simulink model "Experiment_2_cs"  (Simulink 8.4)
settings: Solver=ode5  SolverMode=SingleTasking  StartTime=0.0  StopTime=inf  FixedStep=1/100  RelTol=1e-3
model workspace (MAT data in the model file):
  mbox_table : struct (value not decoded)
  model_closed = 0
  sim_status : num (value not decoded)
PreLoadFcn:
  | mbxruntime.callbacks.PreLoadFcn(bdroot);
PostLoadFcn:
  | mbxruntime.callbacks.PostLoadFcn(bdroot);
InitFcn:
  | mbxruntime.callbacks.InitFcn(bdroot);
StartFcn:
  | mbxruntime.callbacks.StartFcn(bdroot);
StopFcn:
  | mbxruntime.callbacks.StopFcn(bdroot);
undefined symbols (not defined in the file or in its folder): dfreq, gray, InitImageOutputDir, Rec, SDTV, strel, warningInitialVelocity, x0
libraries: simulink x43, PreScanSimulinkLibrary x19, visiontextngfix x15, simulink_extras x11, visionconversions x3, PreScanUsefulBlocks x3, visionsinks x2, visionstatistics x1, visionmorphops x1, visionanalysis x1
(part 1 of 8)
CloseFcn:
  | mbxruntime.callbacks.CloseFcn(bdroot);
settings Model: Creator=PRESCAN  LastModifiedBy=vj-admin
settings OptimizationCC: InitFltsAndDblsToZero=on
settings DebuggingCC: SaveWithParameterizedLinksMsg=none  SignalResolutionControl=TryResolveAllWithWarning  SolverPrmCheckMsg=none  MultiTaskDSMMsg=warning  MultiTaskCondExecSysMsg=none
settings ModelReferenceCC: UpdateModelReferenceTargets=IfOutOfDate
settings SFSimCC: SimParseCustomCode=off
settings SFSimCC: SimCustomHeaderCode=|
  | #include "prescan_collisiondetection_data.h"
  | #include "prescan.h"
  | #include "prescan_platform.h"
  | #include "prescan_v2x_data.h"
settings RTWCC: IncludeERTFirstTime=on
settings GRTTargetCC: TargetFcnLib=ansi_tfl_tmw.mat

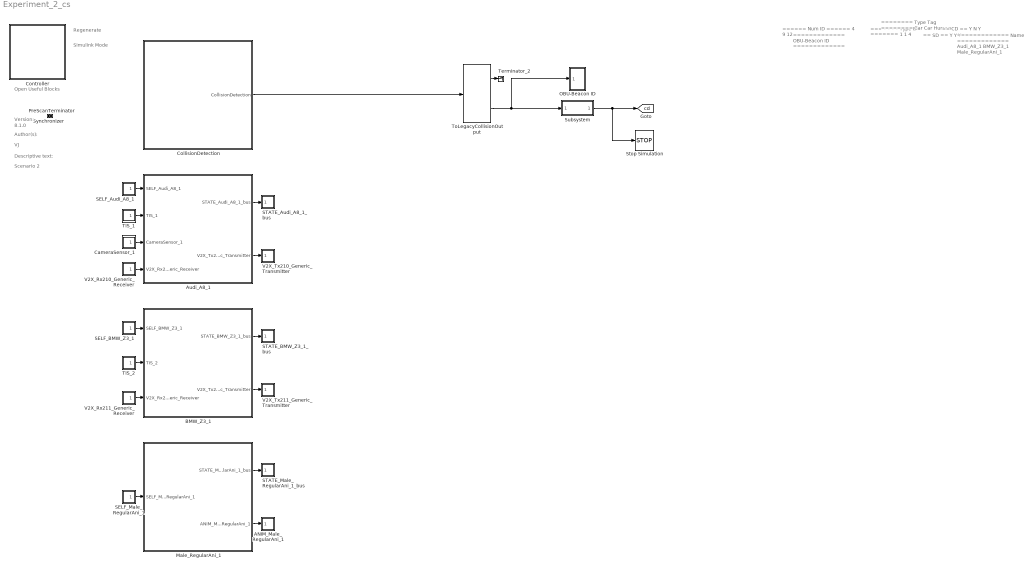
== system Experiment_2_cs ==
  note: Regenerate
  note: Simulink Mode
  note: Open Useful Blocks
  note: 8.1.0
  note: Version:
  note: Author(s):
  note: VJ
  note: Descriptive text:
  note: Scenario 2
  note: ======
      | Num ID
      | ======
      | 4
      | 9
      | 12
  note: =============
      | OBU-Beacon ID
      | =============
  note: =======
      | Type ID
      | =======
      | 1
      | 1
      | 4
  note: ========
      | Type Tag
      | ========
      | Car
      | Car
      | Human
  note: ==
      | SD
      | ==
      | Y
      | Y
      | Y
  note: ==
      | CD
      | ==
      | Y
      | N
      | Y
  note: =============
      | Name
      | =============
      | Audi_A8_1
      | BMW_Z3_1
      | Male_RegularAni_1
  ANIM_Male_RegularAni_1 : Subsystem  Tag=actuator/AnimationOutport  Priority=0  LoadFcn=load('PreScanAnimActuatorData.mat')  Variant=on  OverrideUsingVariant=on  mask(PreScan Sink Block: State Animation){}
      mask help: The Human Animation port allows the human to walk, run or bend
      settings: OpenFcn=open_system([gcb '/ENABLED/Actuator'],'mask')
      mask Help: eval('openHelp(239)')
      mask Display: image(imread('HumanAnimated.jpg'))
  Audi_A8_1 : Subsystem  Tag=WorldObjectSubSystem  InitFcn=UniqueId = '109';  Variant=on  OverrideUsingVariant=on
      mask init:
      | imagePath=which('Audi_A8.jpg');
      settings: OpenFcn=open_system([gcb '/ENABLED'])
      mask Display: image(imread(imagePath));color('white');text(0,0,' ID=4\n')
  BMW_Z3_1 : Subsystem  Tag=WorldObjectSubSystem  InitFcn=UniqueId = '112';  Variant=on  OverrideUsingVariant=on
      mask init:
      | imagePath=which('BMW_Z3.jpg');
      settings: OpenFcn=open_system([gcb '/ENABLED'])
      mask Display: image(imread(imagePath));color('white');text(0,0,' ID=9\n')
  CameraSensor_1 : Subsystem  Tag=sensor/Camera/CameraSensor  Priority=3  Variant=on  OverrideUsingVariant=on  mask(PreScan Source Block: Camera Sensor){}
      mask help: The Camera Sensor provides a color or monochrome image.
      settings: OpenFcn=open_system([gcb '/ENABLED/Sensor'],'mask')
      mask Help: eval('openHelp(457)')
      mask Display: image(imread('CameraSensor.png'))
  CollisionDetection : Subsystem  Tag=sensor/CollisionDetection  Priority=3  LoadFcn=load('PrescanCollisionDetectionData.mat');load('PrescanCollisionDetectionMessage.mat')  Variant=on  OverrideUsingVariant=on  mask(PreScan Source Block: CollisionDetection){}
      mask help: Collision Detection can be used to detect collisions between PreScan components. For Collision Detection the actual component shape is taken into account, so it is not a bounding box approach.
      settings: OpenFcn=open_system([gcb '/ENABLED/Sensor'],'mask')
      mask Help: eval('openHelp(811)')
      mask Display: image(imread('crash.jpg'))
  Controller : Subsystem  Description=FA0A96F99A880E53F0BFF9FE52303144F19899D73F656CE8BF47A1C0F136E2DD  Priority=-1  LoadFcn=load PreScanControllerData  mask(PreScan Simulation Controller){prescanversion='8.1.0', ModelReferencing=off, TimeStep=1/100, ControlMode=0, PreScanExecutionMode=on, ControllerCount=0, ControllerIndex=0, ControllerOptions=''}
      mask prompts: prescanversion "PreScan Version"; ModelReferencing "Use Model Referencing"; TimeStep "Upload Period [s]"; ControlMode "Control Mode"; PreScanExecutionMode "Execution Mode"; ControllerCount "Controller Count"; ControllerIndex "Controller Index"; ControllerOptions "Controller Options"
      mask help:
      | Please do not remove this block from the compilation sheet,
      | as it connects the model to the PreScan environment.
      mask init:
      | model = bdroot(gcb);
      | ExperimentFile = mbxruntime.findExperimentFile(model);
      | 
      | [d1, d2, d3, prescandata] = prescan_Settings();
      | ModelDepo = fullfile(prescandata,'ModelDepo'); 
      | 
      | RTmode = 0;
      | actors = find_system(model,'SearchDepth', 1,'LookUnderMasks', 'all','Tag','WorldObjectSubSystem');
      | for ii=1:length(actors)
      |     actormode = get_param(actors{ii},'OverrideUsingVariant');
      |     if strcmpi(actormode,'off')
      |         RTmode = 1;
      |     end
      | end
      | 
      | SimulationMode = get_param(bdroot,'SimulationMode');
      | if strcmp(SimulationMode, 'rapid-accelerator')
      |     SimulationMode = 'external';
      | end
      | TargetName = get_param(bdroot,'SystemTargetFile');
      settings: ModelCloseFcn=assignin('base',['model_closed_' bdroot],true);
      mask Help: eval('openHelp(812)')
      mask Display: image(imread('prescanlogo.ico'))
  Male_RegularAni_1 : Subsystem  Tag=WorldObjectSubSystem  InitFcn=UniqueId = '116';  Variant=on  OverrideUsingVariant=on
      mask init:
      | imagePath=which('Male_RegularAni.jpg');
      settings: OpenFcn=open_system([gcb '/ENABLED'])
      mask Display: image(imread(imagePath));color('white');text(0,0,' ID=12\n')
  OBU-Beacon ID : Subsystem  Tag=Scope Collision Detections
      settings: DeleteFcn=PreScanBlockDeleteFcn;
      settings: OpenFcn=|
      | blockname=[get_param(gcb,'Parent'),'/',get_param(gcb,'Name')];
      | subblockname=[blockname,'/Collision Detections'];
      | open_system(subblockname);
      | close_system(blockname);
      mask Display:
      | plot([0.5 9.5 9.5 0.5 0.5],[5 5 9 9 5])
      | plot(0,0)
      | plot(10,10)
      | text(0,1,'P+')
  PreScanTerminator : Subsystem  Tag=PreScanTerminator  Priority=999  LoadFcn=load PrescanTerminatorData  mask(PreScan Simulation Terminator){TimeStep=1/100}
      mask prompts: TimeStep "Upload Period [s]"
      mask help:
      | Please do not remove this block from the compilation sheet as it
      | connects the model to the PreScan environment.
      mask Help: eval('openHelp(812)')
      mask Display: image(imread('prescanlogo.ico'))
  SELF_Audi_A8_1 : Subsystem  Tag=sensor/SelfPort  Priority=3  LoadFcn=load('PreScanSelfSensorData.mat')  Variant=on  OverrideUsingVariant=on  mask(PreScan Source Block: SELF){}
      mask help:
      | The SELF port shows (state) information of the actor itself. The outputs are position in the experiment's axis system and the GPS coordinates, and the object's absolute velocity and compass heading.
      |
      | For more information, please click Help.
      settings: OpenFcn=open_system([gcb '/ENABLED/Sensor'],'mask')
      mask Help: eval('openHelp(462)')
      mask Display: image(imread('GPS.png'))
  SELF_BMW_Z3_1 : Subsystem  Tag=sensor/SelfPort  Priority=3  LoadFcn=load('PreScanSelfSensorData.mat')  Variant=on  OverrideUsingVariant=on  mask(PreScan Source Block: SELF){}
      mask help:
      | The SELF port shows (state) information of the actor itself. The outputs are position in the experiment's axis system and the GPS coordinates, and the object's absolute velocity and compass heading.
      |
      | For more information, please click Help.
      settings: OpenFcn=open_system([gcb '/ENABLED/Sensor'],'mask')
      mask Help: eval('openHelp(462)')
      mask Display: image(imread('GPS.png'))
  SELF_Male_RegularAni_1 : Subsystem  Tag=sensor/SelfPort  Priority=3  LoadFcn=load('PreScanSelfSensorData.mat')  Variant=on  OverrideUsingVariant=on  mask(PreScan Source Block: SELF){}
      mask help:
      | The SELF port shows (state) information of the actor itself. The outputs are position in the experiment's axis system and the GPS coordinates, and the object's absolute velocity and compass heading.
      |
      | For more information, please click Help.
      settings: OpenFcn=open_system([gcb '/ENABLED/Sensor'],'mask')
      mask Help: eval('openHelp(462)')
      mask Display: image(imread('GPS.png'))
  STATE_Audi_A8_1_bus : Subsystem  Tag=actuator/StatePort  Priority=0  LoadFcn=load('PreScanStateActuatorData.mat')  Variant=on  OverrideUsingVariant=on  mask(PreScan Sink Block: State){}
      mask help:
      | The Actor State contains a vector signal of size (9x1), containing the following signals:
      |
      | -  Position    	(x,y,z)             	[m]
      | -  Velocity    	(vx,vy,vz)         	[m/s]
      | -  Angles       	(Roll, Pitch, Yaw)	[rad]
      |
      | The Actor state is defined in the global axis system.
      | The state is superponed on the Initial position defined in the GUI.
      |
      | For more information, please click Help.
      settings: OpenFcn=open_system([gcb '/ENABLED/Actuator'],'mask')
      mask Help: eval('openHelp(222)')
      mask Display: image(imread('State.png'))
  STATE_BMW_Z3_1_bus : Subsystem  Tag=actuator/StatePort  Priority=0  LoadFcn=load('PreScanStateActuatorData.mat')  Variant=on  OverrideUsingVariant=on  mask(PreScan Sink Block: State){}
      mask help:
      | The Actor State contains a vector signal of size (9x1), containing the following signals:
      |
      | -  Position    	(x,y,z)             	[m]
      | -  Velocity    	(vx,vy,vz)         	[m/s]
      | -  Angles       	(Roll, Pitch, Yaw)	[rad]
      |
      | The Actor state is defined in the global axis system.
      | The state is superponed on the Initial position defined in the GUI.
      |
      | For more information, please click Help.
      settings: OpenFcn=open_system([gcb '/ENABLED/Actuator'],'mask')
      mask Help: eval('openHelp(222)')
      mask Display: image(imread('State.png'))
  STATE_Male_RegularAni_1_bus : Subsystem  Tag=actuator/StatePort  Priority=0  LoadFcn=load('PreScanStateActuatorData.mat')  Variant=on  OverrideUsingVariant=on  mask(PreScan Sink Block: State){}
      mask help:
      | The Actor State contains a vector signal of size (9x1), containing the following signals:
      |
      | -  Position    	(x,y,z)             	[m]
      | -  Velocity    	(vx,vy,vz)         	[m/s]
      | -  Angles       	(Roll, Pitch, Yaw)	[rad]
      |
      | The Actor state is defined in the global axis system.
      | The state is superponed on the Initial position defined in the GUI.
      |
      | For more information, please click Help.
      settings: OpenFcn=open_system([gcb '/ENABLED/Actuator'],'mask')
      mask Help: eval('openHelp(222)')
      mask Display: image(imread('State.png'))
  Stop Simulation : Stop
  Subsystem : Subsystem
      mask Display: fprintf('CD');
  Synchronizer : Subsystem  Tag=PreScanSynchronizer  Priority=1  LoadFcn=load PrescanSynchronizeData  mask(PreScan Simulation Core Block){TimeStep=1/100}
      mask prompts: TimeStep "Timestep [s]"
      mask help:
      | Please do not remove this block from the PreScan compilation sheet,
      | as it contains essential configuration parameters for a PreScan simulation.
      settings: DeleteFcn=PreScanBlockDeleteFcn;
      mask Display: image(imread('prescanlogo.ico'))
  TIS_1 : Subsystem  Tag=sensor/TIS  Priority=3  LoadFcn=load('PrescanScannerSensorData.mat');load('PrescanScannerSensorMessage.mat')  Variant=on  OverrideUsingVariant=on  mask(PreScan Source Block: Technology Independent Sensor (TIS)){}
      mask help:
      | The Technology Independent Sensor (TIS) provides a sensor with all sensor-related influence factors (like noise, drift and accuracy) without being technology specific (like radar and lidar). The TIS detects the closest point on the geometry of an object.
      |
      | For more information, please click Help.
      settings: OpenFcn=open_system([gcb '/ENABLED/Sensor'],'mask')
      mask Help: eval('openHelp(449)')
      mask Display: image(imread('TIS.png'))
  TIS_2 : Subsystem  Tag=sensor/TIS  Priority=3  LoadFcn=load('PrescanScannerSensorData.mat');load('PrescanScannerSensorMessage.mat')  Variant=on  OverrideUsingVariant=on  mask(PreScan Source Block: Technology Independent Sensor (TIS)){}
      mask help:
      | The Technology Independent Sensor (TIS) provides a sensor with all sensor-related influence factors (like noise, drift and accuracy) without being technology specific (like radar and lidar). The TIS detects the closest point on the geometry of an object.
      |
      | For more information, please click Help.
      settings: OpenFcn=open_system([gcb '/ENABLED/Sensor'],'mask')
      mask Help: eval('openHelp(449)')
      mask Display: image(imread('TIS.png'))
  Terminator_2 : Terminator
  ToLegacyCollisionOutput : PreScanUsefulBlocks/ToLegacyCollisionOutput
  V2X_Rx210_Generic_Receiver : Subsystem  Tag=sensor/plugin/sfun_V2X_Generic_Receiver  Priority=3  Variant=on  OverrideUsingVariant=on  mask(V2X Generic Receiver Block){}
      mask help: V2X Block receiving a Generic message
      settings: OpenFcn=open_system([gcb '/ENABLED/Sensor'],'mask')
      mask Help: eval('openHelp()')
      mask Display: image(imread('V2XR_grayscale.png'))
  V2X_Rx211_Generic_Receiver : Subsystem  Tag=sensor/plugin/sfun_V2X_Generic_Receiver  Priority=3  Variant=on  OverrideUsingVariant=on  mask(V2X Generic Receiver Block){}
      mask help: V2X Block receiving a Generic message
      settings: OpenFcn=open_system([gcb '/ENABLED/Sensor'],'mask')
      mask Help: eval('openHelp()')
      mask Display: image(imread('V2XR_grayscale.png'))
  V2X_Tx210_Generic_Transmitter : Subsystem  Tag=actuator/plugin/sfun_V2X_Generic_Transmitter  Priority=0  Variant=on  OverrideUsingVariant=on  mask(V2X Generic Transmitter Block){}
      mask help: V2X Block transmitting a Generic message
      settings: OpenFcn=open_system([gcb '/ENABLED/Actuator'],'mask')
      mask Help: eval('openHelp()')
      mask Display: image(imread('V2XT_grayscale.png'))
  V2X_Tx211_Generic_Transmitter : Subsystem  Tag=actuator/plugin/sfun_V2X_Generic_Transmitter  Priority=0  Variant=on  OverrideUsingVariant=on  mask(V2X Generic Transmitter Block){}
      mask help: V2X Block transmitting a Generic message
      settings: OpenFcn=open_system([gcb '/ENABLED/Actuator'],'mask')
      mask Help: eval('openHelp()')
      mask Display: image(imread('V2XT_grayscale.png'))
  tag scope: cd=global
  wires:
  CollisionDetection/1(CollisionDetection) -> ToLegacyCollisionOutput/1
  Subsystem/1(cd_out) -> Stop Simulation/1, [cd]
  ToLegacyCollisionOutput/2 -> Subsystem/1(cd_in), OBU-Beacon ID/1(In1)
  ToLegacyCollisionOutput/1 -> Terminator_2/1
  Audi_A8_1/1(STATE_Audi_A8_1_bus) -> STATE_Audi_A8_1_bus/1(STATE_Audi_A8_1_bus)
  SELF_Audi_A8_1/1(SELF_Audi_A8_1) -> Audi_A8_1/1(SELF_Audi_A8_1)
  TIS_1/1(TIS_1) -> Audi_A8_1/2(TIS_1)
  CameraSensor_1/1(CameraSensor_1) -> Audi_A8_1/3(CameraSensor_1)
  Audi_A8_1/2(V2X_Tx210_Generic_Transmitter) -> V2X_Tx210_Generic_Transmitter/1(V2X_Tx210_Generic_Transmitter)
  V2X_Rx210_Generic_Receiver/1(V2X_Rx210_Generic_Receiver) -> Audi_A8_1/4(V2X_Rx210_Generic_Receiver)
  BMW_Z3_1/1(STATE_BMW_Z3_1_bus) -> STATE_BMW_Z3_1_bus/1(STATE_BMW_Z3_1_bus)
  SELF_BMW_Z3_1/1(SELF_BMW_Z3_1) -> BMW_Z3_1/1(SELF_BMW_Z3_1)
  TIS_2/1(TIS_2) -> BMW_Z3_1/2(TIS_2)
  BMW_Z3_1/2(V2X_Tx211_Generic_Transmitter) -> V2X_Tx211_Generic_Transmitter/1(V2X_Tx211_Generic_Transmitter)
  V2X_Rx211_Generic_Receiver/1(V2X_Rx211_Generic_Receiver) -> BMW_Z3_1/3(V2X_Rx211_Generic_Receiver)
  Male_RegularAni_1/1(STATE_Male_RegularAni_1_bus) -> STATE_Male_RegularAni_1_bus/1(STATE_Male_RegularAni_1_bus)
  Male_RegularAni_1/2(ANIM_Male_RegularAni_1) -> ANIM_Male_RegularAni_1/1(ANIM_Male_RegularAni_1)
  SELF_Male_RegularAni_1/1(SELF_Male_RegularAni_1) -> Male_RegularAni_1/1(SELF_Male_RegularAni_1)

== system Experiment_2_cs/ANIM_Male_RegularAni_1 ==
  ANIM_Male_RegularAni_1 : Inport  Tag=inport/AnimationOutport  OutDataTypeStr=Bus: PRESCAN_ANIMACTUATORDATA  PortDimensions=1  SampleTime=1/100  BusOutputAsStruct=on
  DISABLED : Subsystem  VariantControl=off
  ENABLED : Subsystem  VariantControl=on

== system Experiment_2_cs/Audi_A8_1 ==
  SELF_Audi_A8_1 : Inport  Tag=inport/SelfPort  OutDataTypeStr=Bus: PRESCAN_SELFSENSORDATA  PortDimensions=1  SampleTime=1/100  BusOutputAsStruct=on
  TIS_1 : Inport  Tag=inport/TIS  Port=2  OutDataTypeStr=Bus: PRESCAN_SCANNERSENSOR_MESSAGE  PortDimensions=3  SampleTime=1/50  BusOutputAsStruct=on
  CameraSensor_1 : Inport  Tag=inport/Camera/CameraSensor  Port=3  OutDataTypeStr=uint8  SampleTime=1/50  BusOutputAsStruct=on
  V2X_Rx210_Generic_Receiver : Inport  Tag=inport/plugin/sfun_V2X_Generic_Receiver  Port=4  BusOutputAsStruct=on
  DISABLED : Subsystem  VariantControl=off
  ENABLED : Subsystem  VariantControl=on
  STATE_Audi_A8_1_bus : Outport  Tag=outport/StatePort  OutDataTypeStr=Bus: PRESCAN_STATEACTUATORDATA  PortDimensions=1  SampleTime=1/100
  V2X_Tx210_Generic_Transmitter : Outport  Tag=outport/plugin/sfun_V2X_Generic_Transmitter  Port=2

== system Experiment_2_cs/BMW_Z3_1 ==
  SELF_BMW_Z3_1 : Inport  Tag=inport/SelfPort  OutDataTypeStr=Bus: PRESCAN_SELFSENSORDATA  PortDimensions=1  SampleTime=1/100  BusOutputAsStruct=on
  TIS_2 : Inport  Tag=inport/TIS  Port=2  OutDataTypeStr=Bus: PRESCAN_SCANNERSENSOR_MESSAGE  PortDimensions=3  SampleTime=1/50  BusOutputAsStruct=on
  V2X_Rx211_Generic_Receiver : Inport  Tag=inport/plugin/sfun_V2X_Generic_Receiver  Port=3  BusOutputAsStruct=on
  DISABLED : Subsystem  VariantControl=off
  ENABLED : Subsystem  VariantControl=on
  STATE_BMW_Z3_1_bus : Outport  Tag=outport/StatePort  OutDataTypeStr=Bus: PRESCAN_STATEACTUATORDATA  PortDimensions=1  SampleTime=1/100
  V2X_Tx211_Generic_Transmitter : Outport  Tag=outport/plugin/sfun_V2X_Generic_Transmitter  Port=2

== system Experiment_2_cs/CameraSensor_1 ==
  DISABLED : Subsystem  VariantControl=off
  ENABLED : Subsystem  VariantControl=on
  CameraSensor_1 : Outport  Tag=outport/Camera/CameraSensor  OutDataTypeStr=uint8  SampleTime=1/50

== system Experiment_2_cs/CollisionDetection ==
  DISABLED : Subsystem  VariantControl=off
  ENABLED : Subsystem  VariantControl=on
  CollisionDetection : Outport  Tag=outport/CollisionDetection  OutDataTypeStr=Bus: PRESCAN_COLLISIONDETECTION_MESSAGE  PortDimensions=5  SampleTime=1/100

== system Experiment_2_cs/Controller ==
  Terminator : Terminator
  sfun_Controller : S-Function  FunctionName=sfun_Controller  Parameters=SParameter1, SParameter2, SParameter3, SParameter4, SParameter5, SParameter6, SParameter7, SParameter8, SParameter9, SParameter10, SampleTime  EnableBusSupport=off  mask(Legacy Function){SFunctionSpec=void prescan_outputFcn(void** work1, PRESCAN_CONTROLLERDATA y1[1]), SParameter1=uint8([ExperimentFile 0]), SParameter2=uint8([ModelDepo 0]), SParameter3=uint8([ControllerOptions 0]), SParameter4=RTmode, SParameter5=PreScanExecutionMode, SParameter6=ControlMode, SParameter7=ControllerCount, SParameter8=ControllerIndex, SParameter9=uint8([SimulationMode 0]), SParameter10=uint8([TargetName 0]), SampleTime=TimeStep, ShowSpec=on}
      mask prompts: SParameter1 "P1:"; SParameter2 "P2:"; SParameter3 "P3:"; SParameter4 "P4:"; SParameter5 "P5:"; SParameter6 "P6:"; SParameter7 "P7:"; SParameter8 "P8:"; SParameter9 "P9:"; SParameter10 "P10:"; SampleTime "Sample time (-1 for inherited):"; ShowSpec "Display function specification"
      mask help:
      | This block allows you to call the legacy functions specified by the following Legacy Code Tool definition:
      | def.SFunctionName = 'sfun_Controller';
      | def.OutputFcnSpec = 'void prescan_outputFcn(void** work1, PRESCAN_CONTROLLERDATA y1[1])';
      | def.StartFcnSpec = 'void prescan_startFcn(void ** work1, uint8 p1[], uint8 p2[], uint8 p3[], double p4, double p5, double p6, double p7, double p8, uint8 p9[], uint8 p10[])';
      | def.TerminateFcnSpec = 'void prescan_terminateFcn(void** work1)';
      | def.HeaderFiles = {'prescan_controller_data.h', 'prescan_SFunLibrary.h', 'prescan_LogHandler.h', 'prescan_CreateLogHandler.h', 'prescan_ErrorHandler.h', 'prescan_CreateErrorHandler.h', 'prescan_modify.h', 'ModuleDLL.h'};
      | def.SourceFiles = {'prescan_MexLogHandler.cpp', 'prescan_SimStructErrorHandler.cpp', 'prescan_LogHandler.cpp', 'prescan_ErrorHandler.cpp', 'prescan_Modify.cpp'};
      | def.HostLibFiles = {'sensorinterfaced.lib'};
      | def.TargetLibFiles = {'sensorinterfaced.so'};
      | def.IncPaths = {'.', 'C:\projects\prescan\rt_vislibrary\vis\..\pimp\include\sensors\InterfaceRTW'};
      | def.SrcPaths = {'C:\projects\prescan\rt_vislibrary\vis\..\pimp\include\sensors\InterfaceRTW', 'C:\projects\prescan\rt_vislibrary\vis\..\pimp\include\sensors\InterfaceRTW\ccurrt'};
      | def.LibPaths = {'C:\\projects\\prescan\\vislibrary_build\lib'};
      | def.SampleTime = 'parameterized';
      mask Help: <p>This block was generated automatically by the Legacy Code Tool. For detailed help on this tool, call<a href="matlab:legacy_code('help')"> legacy_code('help')</a>.</p>
      mask Callback ShowSpec:
      | if strcmp(get_param(gcbh, 'ShowSpec'), 'on')
      |   set_param(gcbh, 'MaskDisplay', sprintf('fprintf(''%s'');', get_param(gcbh, 'SFunctionSpec')));
      | else
      |   set_param(gcbh, 'MaskDisplay', sprintf('fprintf(''%s'');', get_param(gcbh, 'FunctionName')));
      | end
      mask Display: fprintf('void prescan_outputFcn(void** work1, PRESCAN_CONTROLLERDATA y1[1])');
  wires:
  sfun_Controller/1 -> Terminator/1

== system Experiment_2_cs/Male_RegularAni_1 ==
  SELF_Male_RegularAni_1 : Inport  Tag=inport/SelfPort  OutDataTypeStr=Bus: PRESCAN_SELFSENSORDATA  PortDimensions=1  SampleTime=1/100  BusOutputAsStruct=on
  DISABLED : Subsystem  VariantControl=off
  ENABLED : Subsystem  VariantControl=on
  STATE_Male_RegularAni_1_bus : Outport  Tag=outport/StatePort  OutDataTypeStr=Bus: PRESCAN_STATEACTUATORDATA  PortDimensions=1  SampleTime=1/100
  ANIM_Male_RegularAni_1 : Outport  Tag=outport/AnimationOutport  Port=2  OutDataTypeStr=Bus: PRESCAN_ANIMACTUATORDATA  PortDimensions=1  SampleTime=1/100

== system Experiment_2_cs/OBU-Beacon ID ==
  In1 : Inport
  Collision Detections : Scope  NumInputPorts=5
      settings: YMin=0~0~0~0~0  YMax=10~10~10~10~10  SaveName=ScopeData2
  Demux2 : Demux  Outputs=5
  wires:
  In1/1 -> Demux2/1
  Demux2/5 -> Collision Detections/5
  Demux2/4 -> Collision Detections/4
  Demux2/3 -> Collision Detections/3
  Demux2/2 -> Collision Detections/2
  Demux2/1 -> Collision Detections/1

== system Experiment_2_cs/PreScanTerminator ==
  Terminator : Terminator
  sfun_Terminator : S-Function  FunctionName=sfun_Terminator  Parameters=SampleTime  EnableBusSupport=off  mask(Legacy Function){SFunctionSpec=void prescan_terminator_outputFcn(void ** work1, PRESCAN_TERMINATORDATA y1[1]), SampleTime=TimeStep, ShowSpec=on}
      mask prompts: SampleTime "Sample time (-1 for inherited):"; ShowSpec "Display function specification"
      mask help:
      | This block allows you to call the legacy functions specified by the following Legacy Code Tool definition:
      | def.SFunctionName = 'sfun_Terminator';
      | def.OutputFcnSpec = 'void prescan_terminator_outputFcn(void ** work1, PRESCAN_TERMINATORDATA y1[1])';
      | def.StartFcnSpec = 'void prescan_terminator_startFcn(void ** work1)';
      | def.TerminateFcnSpec = 'void prescan_terminator_terminateFcn(void ** work1)';
      | def.HeaderFiles = {'prescan_terminator_data.h'};
      | def.HostLibFiles = {'sensorinterfaced.lib'};
      | def.IncPaths = {'src', 'C:\prescandev\vislibrary\vis\..\pimp\include\sensors\InterfaceRTW'};
      | def.SrcPaths = {'src'};
      | def.LibPaths = {'C:\\prescandev\\vislibrary_build\lib'};
      | def.SampleTime = 'parameterized';
      | def.Options.language = 'C++';
      mask Help: <p>This block was generated automatically by the Legacy Code Tool. For detailed help on this tool, call<a href="matlab:legacy_code('help')"> legacy_code('help')</a>.</p>
      mask Callback ShowSpec:
      | if strcmp(get_param(gcbh, 'ShowSpec'), 'on')
      |   set_param(gcbh, 'MaskDisplay', sprintf('fprintf(''%s'');', get_param(gcbh, 'SFunctionSpec')));
      | else
      |   set_param(gcbh, 'MaskDisplay', sprintf('fprintf(''%s'');', get_param(gcbh, 'FunctionName')));
      | end
      mask Display: fprintf('void prescan_terminator_outputFcn(void ** work1, PRESCAN_TERMINATORDATA y1[1])');
  wires:
  sfun_Terminator/1 -> Terminator/1

== system Experiment_2_cs/SELF_Audi_A8_1 ==
  DISABLED : Subsystem  VariantControl=off
  ENABLED : Subsystem  VariantControl=on
  SELF_Audi_A8_1 : Outport  Tag=outport/SelfPort  OutDataTypeStr=Bus: PRESCAN_SELFSENSORDATA  PortDimensions=1  SampleTime=1/100

== system Experiment_2_cs/SELF_BMW_Z3_1 ==
  DISABLED : Subsystem  VariantControl=off
  ENABLED : Subsystem  VariantControl=on
  SELF_BMW_Z3_1 : Outport  Tag=outport/SelfPort  OutDataTypeStr=Bus: PRESCAN_SELFSENSORDATA  PortDimensions=1  SampleTime=1/100

== system Experiment_2_cs/SELF_Male_RegularAni_1 ==
  DISABLED : Subsystem  VariantControl=off
  ENABLED : Subsystem  VariantControl=on
  SELF_Male_RegularAni_1 : Outport  Tag=outport/SelfPort  OutDataTypeStr=Bus: PRESCAN_SELFSENSORDATA  PortDimensions=1  SampleTime=1/100

== system Experiment_2_cs/STATE_Audi_A8_1_bus ==
  STATE_Audi_A8_1_bus : Inport  Tag=inport/StatePort  OutDataTypeStr=Bus: PRESCAN_STATEACTUATORDATA  PortDimensions=1  SampleTime=1/100  BusOutputAsStruct=on
  DISABLED : Subsystem  VariantControl=off
  ENABLED : Subsystem  VariantControl=on

== system Experiment_2_cs/STATE_BMW_Z3_1_bus ==
  STATE_BMW_Z3_1_bus : Inport  Tag=inport/StatePort  OutDataTypeStr=Bus: PRESCAN_STATEACTUATORDATA  PortDimensions=1  SampleTime=1/100  BusOutputAsStruct=on
  DISABLED : Subsystem  VariantControl=off
  ENABLED : Subsystem  VariantControl=on

== system Experiment_2_cs/STATE_Male_RegularAni_1_bus ==
  STATE_Male_RegularAni_1_bus : Inport  Tag=inport/StatePort  OutDataTypeStr=Bus: PRESCAN_STATEACTUATORDATA  PortDimensions=1  SampleTime=1/100  BusOutputAsStruct=on
  DISABLED : Subsystem  VariantControl=off
  ENABLED : Subsystem  VariantControl=on

== system Experiment_2_cs/Subsystem ==
  cd_in : Inport
  Integer Delay : Delay  DelayLength=1  InputProcessing=Inherited
  Logical Operator : Logic  AllPortsSameDT=off  OutDataTypeStr=boolean
  cd_out : Outport
  wires:
  cd_in/1 -> Integer Delay/1, Logical Operator/1
  Logical Operator/1 -> cd_out/1
  Integer Delay/1 -> Logical Operator/2

== system Experiment_2_cs/Synchronizer ==
  Bus Selector1 : BusSelector  OutputSignals=FederateStopped
  Stop Simulation : Stop
  sfun_Synchronizer : S-Function  FunctionName=sfun_Synchronizer  Parameters=SampleTime  EnableBusSupport=off  mask(Legacy Function){SFunctionSpec=void prescan_synchronizer_outputFcn(void ** work1, PRESCAN_SYNCHRONIZEDATA y1[1]), SampleTime=TimeStep, ShowSpec=on}
      mask prompts: SampleTime "Sample time (-1 for inherited):"; ShowSpec "Display function specification"
      mask help:
      | This block allows you to call the legacy functions specified by the following Legacy Code Tool definition:
      | def.SFunctionName = 'sfun_Synchronizer';
      | def.OutputFcnSpec = 'void prescan_synchronizer_outputFcn(void ** work1, PRESCAN_SYNCHRONIZEDATA y1[1])';
      | def.StartFcnSpec = 'void prescan_synchronizer_startFcn(void ** work1)';
      | def.TerminateFcnSpec = 'void prescan_synchronizer_terminateFcn(void ** work1)';
      | def.HeaderFiles = {'prescan_synchronizer_data.h'};
      | def.HostLibFiles = {'sensorinterfaced.lib'};
      | def.IncPaths = {'src', 'C:\prescandev\vislibrary\vis\..\pimp\include\sensors\InterfaceRTW'};
      | def.SrcPaths = {'src'};
      | def.LibPaths = {'C:\\prescandev\\vislibrary_build\lib'};
      | def.SampleTime = 'parameterized';
      | def.Options.language = 'C++';
      mask Help: <p>This block was generated automatically by the Legacy Code Tool. For detailed help on this tool, call<a href="matlab:legacy_code('help')"> legacy_code('help')</a>.</p>
      mask Callback ShowSpec:
      | if strcmp(get_param(gcbh, 'ShowSpec'), 'on')
      |   set_param(gcbh, 'MaskDisplay', sprintf('fprintf(''%s'');', get_param(gcbh, 'SFunctionSpec')));
      | else
      |   set_param(gcbh, 'MaskDisplay', sprintf('fprintf(''%s'');', get_param(gcbh, 'FunctionName')));
      | end
      mask Display: fprintf('void prescan_synchronizer_outputFcn(void ** work1, PRESCAN_SYNCHRONIZEDATA y1[1])');
  wires:
  Bus Selector1/1 -> Stop Simulation/1  "<FederateStopped>"
  sfun_Synchronizer/1 -> Bus Selector1/1

== system Experiment_2_cs/TIS_1 ==
  DISABLED : Subsystem  VariantControl=off
  ENABLED : Subsystem  VariantControl=on
  TIS_1 : Outport  Tag=outport/TIS  OutDataTypeStr=Bus: PRESCAN_SCANNERSENSOR_MESSAGE  PortDimensions=3  SampleTime=1/50

== system Experiment_2_cs/TIS_2 ==
  DISABLED : Subsystem  VariantControl=off
  ENABLED : Subsystem  VariantControl=on
  TIS_2 : Outport  Tag=outport/TIS  OutDataTypeStr=Bus: PRESCAN_SCANNERSENSOR_MESSAGE  PortDimensions=3  SampleTime=1/50

== system Experiment_2_cs/V2X_Rx210_Generic_Receiver ==
  DISABLED : Subsystem  VariantControl=off
  ENABLED : Subsystem  VariantControl=on
  V2X_Rx210_Generic_Receiver : Outport  Tag=outport/plugin/sfun_V2X_Generic_Receiver

== system Experiment_2_cs/V2X_Rx211_Generic_Receiver ==
  DISABLED : Subsystem  VariantControl=off
  ENABLED : Subsystem  VariantControl=on
  V2X_Rx211_Generic_Receiver : Outport  Tag=outport/plugin/sfun_V2X_Generic_Receiver

== system Experiment_2_cs/V2X_Tx210_Generic_Transmitter ==
  V2X_Tx210_Generic_Transmitter : Inport  Tag=inport/plugin/sfun_V2X_Generic_Transmitter  BusOutputAsStruct=on
  DISABLED : Subsystem  VariantControl=off
  ENABLED : Subsystem  VariantControl=on

== system Experiment_2_cs/V2X_Tx211_Generic_Transmitter ==
  V2X_Tx211_Generic_Transmitter : Inport  Tag=inport/plugin/sfun_V2X_Generic_Transmitter  BusOutputAsStruct=on
  DISABLED : Subsystem  VariantControl=off
  ENABLED : Subsystem  VariantControl=on

== system Experiment_2_cs/ANIM_Male_RegularAni_1/DISABLED ==
  ANIM_Male_RegularAni_1 : Inport  Tag=inport/AnimationOutport  OutDataTypeStr=Bus: PRESCAN_ANIMACTUATORDATA  PortDimensions=1  SampleTime=1/100  BusOutputAsStruct=on
  TRM1 : Terminator
  wires:
  ANIM_Male_RegularAni_1/1 -> TRM1/1

== system Experiment_2_cs/ANIM_Male_RegularAni_1/ENABLED ==
  ANIM_Male_RegularAni_1 : Inport  Tag=inport/AnimationOutport  OutDataTypeStr=Bus: PRESCAN_ANIMACTUATORDATA  PortDimensions=1  SampleTime=1/100  BusOutputAsStruct=on
  Actuator : S-Function  FunctionName=sfun_AnimActuator  Parameters=UniqueID, TimeStep  EnableBusSupport=off  mask(PreScan Sink Block: State Animation){UniqueID=116, TimeStep=1/100}
      mask prompts: UniqueID "Auto-Assigned: Unique ID"; TimeStep "Auto-Assigned: Upload Period [s]"
      mask help: The Human Animation port allows the human to walk, run or bend
      mask Help: eval('openHelp(239)')
      mask Display: image(imread('HumanAnimated.jpg'))
  wires:
  ANIM_Male_RegularAni_1/1 -> Actuator/1

== system Experiment_2_cs/Audi_A8_1/DISABLED ==
  SELF_Audi_A8_1 : Inport  Tag=inport/SelfPort  OutDataTypeStr=Bus: PRESCAN_SELFSENSORDATA  PortDimensions=1  SampleTime=1/100  BusOutputAsStruct=on
  TIS_1 : Inport  Tag=inport/TIS  Port=2  OutDataTypeStr=Bus: PRESCAN_SCANNERSENSOR_MESSAGE  PortDimensions=3  SampleTime=1/50  BusOutputAsStruct=on
  CameraSensor_1 : Inport  Tag=inport/Camera/CameraSensor  Port=3  OutDataTypeStr=uint8  SampleTime=1/50  BusOutputAsStruct=on
  V2X_Rx210_Generic_Receiver : Inport  Tag=inport/plugin/sfun_V2X_Generic_Receiver  Port=4  BusOutputAsStruct=on
  GND1 : Subsystem
  GND2 : Ground
  TRM{1..4} (4 alike) : Terminator
  STATE_Audi_A8_1_bus : Outport  Tag=outport/StatePort  OutDataTypeStr=Bus: PRESCAN_STATEACTUATORDATA  PortDimensions=1  SampleTime=1/100
  V2X_Tx210_Generic_Transmitter : Outport  Tag=outport/plugin/sfun_V2X_Generic_Transmitter  Port=2
  wires:
  SELF_Audi_A8_1/1 -> TRM1/1
  TIS_1/1 -> TRM2/1
  CameraSensor_1/1 -> TRM3/1
  V2X_Rx210_Generic_Receiver/1 -> TRM4/1
  GND1/1(bus) -> STATE_Audi_A8_1_bus/1
  GND2/1 -> V2X_Tx210_Generic_Transmitter/1
